simulink model "ec01m_ethercat_master_sldrt"  (R2025b)
settings: Solver=FixedStepDiscrete  StartTime=0.0  StopTime=100  FixedStep=0.05  RelTol=1e-3  EnableMultiTasking=on
libraries: slrealtimeutilitieslib x2, sldrtlib x1
settings Model: FPTRunName=Active  ExtModeTrigDuration=2  Creator=ihout  LastModifiedBy=ihout
settings SolverCC: AlgebraicLoopSolver=TrustRegion  PositivePriorityOrder=on
settings DataIOCC: LimitDataPoints=on  SaveFormat=Array  ReturnWorkspaceOutputs=off
settings OptimizationCC: DefaultParameterBehavior=Inlined  EnhancedBackFolding=on  PassReuseOutputArgsThreshold=0.0  ExpressionDepthLimit=2147483647.0  MaxStackSize=64  SimCompilerOptimization=on  OptimizeBlockOrder=speed  DifferentSizesBufferReuse=on  OptimizationCustomize=off
settings DebuggingCC: UnderspecifiedInitializationDetection=Classic  MergeDetectMultiDrivingBlocksExec=none  ParameterTunabilityLossMsg=error  FcnCallInpInsideContextMsg=warning  UnconnectedInputMsg=warning  UnconnectedOutputMsg=warning  UnconnectedLineMsg=warning  AllowSymbolicDim=off  StateNameClashWarn=warning  SFUnexpectedBacktrackingDiag=warning  SFNoUnconditionalDefaultTransitionDiag=warning  SFExecutionAtInitializationDiag=none  ArithmeticOperatorsInVariantConditions=warning
settings HardwareCC: ProdBitPerLong=64.0  ProdHWDeviceType=Intel->x86-64 (Linux 64)  UseEmbeddedCoderFeatures=off  UseSimulinkCoderFeatures=off
settings ModelReferenceCC: EnableRefExpFcnMdlSchedulingChecks=on  PropagateSignalLabelsOutOfModel=off
settings SFSimCC: SimUseLocalCustomCode=off  MATLABDynamicMemAlloc=off  CustomCodeUndefinedFunction=UseInterfaceOnly
settings RTWCC: SystemTargetFile=sldrt.tlc  TemplateMakefile=sldrt.tmf  GenerateReport=on  RTWVerbose=off  RTWUseLocalCustomCode=off  BuildConfiguration=Faster Runs  LaunchReport=on  RTWCompilerOptimization=on  GPUComputeCapability=3.5  Description=Simulink Desktop Real-Time
settings CodeAppCC: ForceParamTrailComments=on  MaxIdLength=95.0  OperatorAnnotations=on
settings SimulinkDesktopRealTimeCC: ExtModeTransport=0.0  ExtModeStaticAllocSize=1000000.0  TargetLibSuffix=_sldrt.a  TargetPreCompLibLocation=C:\Program Files\MATLAB\R2025b\toolbox\sldrt\lib\win64  TargetLangStandard=C89/C90 (ANSI)  MultiwordLength=2048.0  DynamicStringBufferSize=256.0  ParMdlRefBuildCompliant=on  PreserveMATLABNamespacesInGeneratedCode=on  SubcomponentCodeInterfacePackaging=Reusable function
settings ConfigComp: CovMetricSettings=dw  CovSaveCumulativeToWorkspaceVar=on  CovSaveSingleToWorkspaceVar=on  CovExternalEMLEnable=off  CovSFcnEnable=off

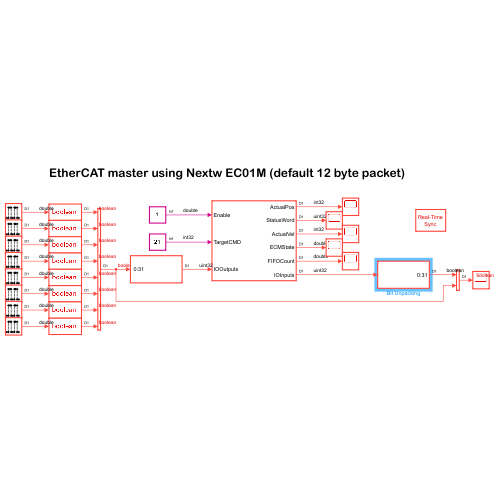
[thumbnail: Simulink's stored preview of the top-level diagram]
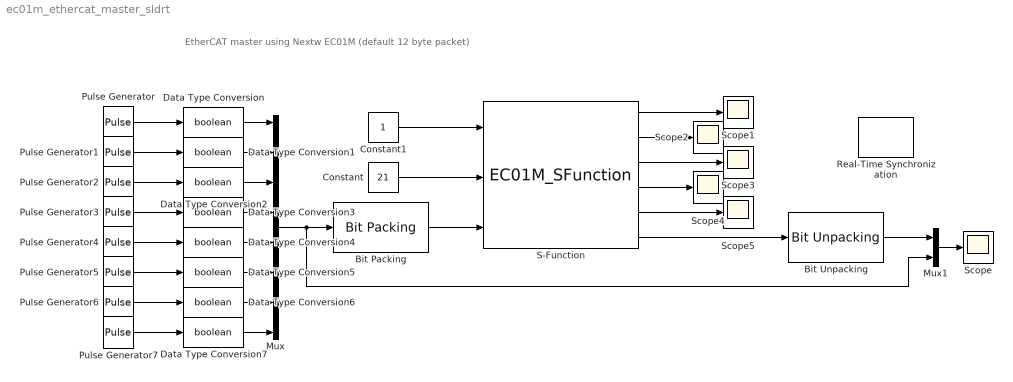
== system ec01m_ethercat_master_sldrt ==
  note: EtherCAT master using Nextw EC01M (default 12 byte packet)
  Bit Packing : slrealtimeutilitieslib/Bit Packing  MaskBitPatterns={[0:31]}  MaskPackDataType=uint32  MaskPackDataSize=[1]
  Bit Unpacking : slrealtimeutilitieslib/Bit Unpacking  SignExtend=on  MaskBitPatterns={[0:31]}  MaskPackDataType=uint32  MaskPackDataSize=[1]  MaskUnpackDataTypes={'boolean'}  MaskUnpackDataSizes={[32]}
  Constant : Constant  Value=21  OutDataTypeStr=int32
  Constant1 : Constant  OutDataTypeStr=double
  Data Type Conversion{,1..7} (8 alike) : DataTypeConversion  OutDataTypeStr=boolean  SaturateOnIntegerOverflow=off  RndMeth=Floor
  Mux : Mux  Inputs=8
  Mux1 : Mux  Inputs=2
  Pulse Generator{,1..7} (8 alike) : DiscretePulseGenerator  Period=10  PulseWidth=5  SampleTime=0.05
  Real-Time Synchronization : sldrtlib/Real-Time Synchronization  SampleTime=0.05  MaxMissedTicks=100  ShowMissedTicks=off  YieldWhenWaiting=off
  S-Function : S-Function  FunctionName=EC01M_SFunction  Parameters=num_slaves,slave_types,drive_mode,sync_mode,dc_cycle_us,sample_time,io_refresh  SFunctionModules='NEXTWUSBLib'  SFunctionDeploymentMode=off  EnableBusSupport=off  mask{num_slaves=1, slave_types=1, drive_mode=CSP, sync_mode=FREERUN, dc_cycle_us=2000, sample_time=0.05, io_refresh=100}
      mask prompts: num_slaves "Number of Slaves"; slave_types "Slave Types (0-DRIVE, 1-IO, 2-HSP ,3-STEP, 15-NONE)"; drive_mode "Drive Mode"; sync_mode "Synchonization Mode"; dc_cycle_us "DC Cycle"; sample_time "Sample Time"; io_refresh "IO Refresh"
      mask Display:
      | port_label('input',1,'Enable');
      | port_label('input',2,'TargetCMD');
      | port_label('input',3,'IOOutputs');
      | 
      | port_label('output',1,'ActualPos');
      | port_label('output',2,'StatusWord');
      | port_label('output',3,'ActualVel');
      | port_label('output',4,'ECMState');
      | port_label('output',5,'FIFOCount');
      | port_label('output',6,'IOInputs');
  Scope{,1..5} (6 alike) : Scope
      Scope settings: ActiveDisplayYMinimum=-2.125  ActiveDisplayYMaximum=9.125
      Scope1 settings: ActiveDisplayYMinimum=3.5  ActiveDisplayYMaximum=8.5
      Scope2 settings: ActiveDisplayYMinimum=3.5  ActiveDisplayYMaximum=8.5  DataLoggingVariableName=ScopeData2
      Scope3 settings: ActiveDisplayYMinimum=3.5  ActiveDisplayYMaximum=8.5  DataLoggingVariableName=ScopeData3
      Scope4 settings: ActiveDisplayYMinimum=3.5  ActiveDisplayYMaximum=8.5  DataLoggingVariableName=ScopeData4
      Scope5 settings: ActiveDisplayYMinimum=3.5  ActiveDisplayYMaximum=8.5  DataLoggingVariableName=ScopeData5
  wires:
  Mux/1 -> Mux1/2, Bit Packing/1
  Mux1/1 -> Scope/1
  Data Type Conversion/1 -> Mux/1
  Data Type Conversion6/1 -> Mux/7
  Data Type Conversion5/1 -> Mux/6
  Data Type Conversion7/1 -> Mux/8
  Data Type Conversion2/1 -> Mux/3
  Data Type Conversion3/1 -> Mux/4
  Data Type Conversion4/1 -> Mux/5
  Data Type Conversion1/1 -> Mux/2
  S-Function/6 -> Bit Unpacking/1
  Bit Packing/1 -> S-Function/3
  Pulse Generator/1 -> Data Type Conversion/1
  Pulse Generator1/1 -> Data Type Conversion1/1
  Pulse Generator2/1 -> Data Type Conversion2/1
  Pulse Generator4/1 -> Data Type Conversion4/1
  Pulse Generator3/1 -> Data Type Conversion3/1
  Pulse Generator5/1 -> Data Type Conversion5/1
  Pulse Generator7/1 -> Data Type Conversion7/1
  Pulse Generator6/1 -> Data Type Conversion6/1
  Bit Unpacking/1 -> Mux1/1
  S-Function/1 -> Scope1/1
  S-Function/2 -> Scope2/1
  S-Function/3 -> Scope3/1
  S-Function/4 -> Scope4/1
  S-Function/5 -> Scope5/1
  Constant1/1 -> S-Function/1
  Constant/1 -> S-Function/2
